simulink model "Ex_3"  (Simulink 8.0)
settings: Solver=ode45  StartTime=0.0  StopTime=10.0  RelTol=1e-3
settings Model: Creator=Faradars  LastModifiedBy=Faradars

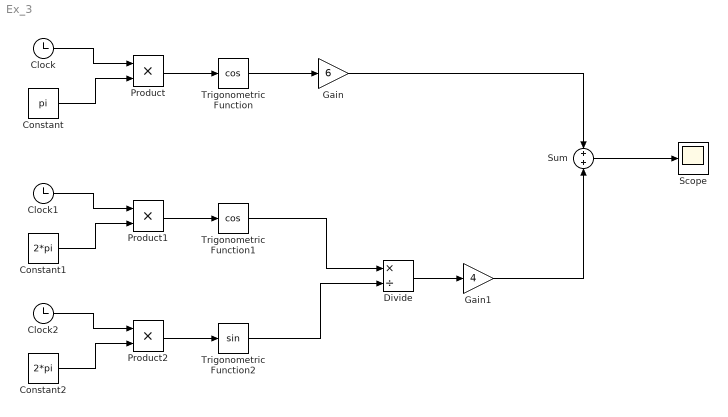
== system Ex_3 ==
  Clock : Clock
  Clock1 : Clock
  Clock2 : Clock
  Constant : Constant  Value=pi
  Constant1 : Constant  Value=2*pi
  Constant2 : Constant  Value=2*pi
  Divide : Product  Inputs=*/
  Gain : Gain  Gain=6
  Gain1 : Gain  Gain=4
  Product : Product  RndMeth=Zero
  Product1 : Product  RndMeth=Zero
  Product2 : Product  RndMeth=Zero
  Scope : Scope
  Sum : Sum  Inputs=+|+
  Trigonometric Function : Trigonometry  Operator=cos
  Trigonometric Function1 : Trigonometry  Operator=cos
  Trigonometric Function2 : Trigonometry
  wires:
  Product/1 -> Trigonometric Function/1
  Clock/1 -> Product/1
  Constant/1 -> Product/2
  Trigonometric Function/1 -> Gain/1
  Product1/1 -> Trigonometric Function1/1
  Clock1/1 -> Product1/1
  Constant1/1 -> Product1/2
  Trigonometric Function1/1 -> Divide/1
  Product2/1 -> Trigonometric Function2/1
  Clock2/1 -> Product2/1
  Constant2/1 -> Product2/2
  Trigonometric Function2/1 -> Divide/2
  Divide/1 -> Gain1/1
  Gain1/1 -> Sum/2
  Gain/1 -> Sum/1
  Sum/1 -> Scope/1
